simulink model "EE382lab51"  (R2016a)
settings: Solver=VariableStepAuto  StartTime=0.0  StopTime=1.0  RelTol=1e-3
settings Model: Creator=Tryrant  LastModifiedBy=Tryrant

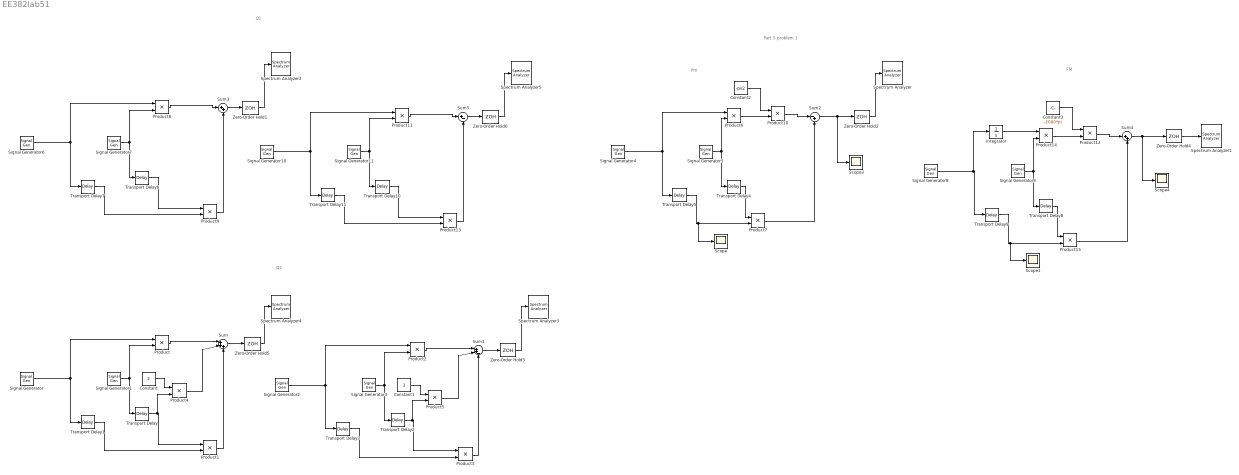
== system EE382lab51 ==
  note: Part 5 problem 1
  note: Q2
  note: Q1
  note: FM
  note: Pm
  Constant : Constant  Value=2
  Constant1 : Constant  Value=2
  Constant2 : Constant  Value=-pi/2
  Constant3 : Constant  Value=-2000*pi
  Integrator : Integrator
  Product{,1..15} (16 alike) : Product
  Scope{,1,3..4} (4 alike) : Scope
  Signal Generator{,1..3,6..7,10..11} (8 alike) : SignalGenerator  Frequency=10000
  Signal Generator4 : SignalGenerator  WaveForm=sawtooth  Frequency=1000
  Signal Generator5 : SignalGenerator  Amplitude=2  Frequency=2*pi*10^6
  Signal Generator8 : SignalGenerator  WaveForm=sawtooth  Frequency=1000
  Signal Generator9 : SignalGenerator  Amplitude=2  Frequency=2*pi*10^6  Units=rad/sec
  Spectrum Analyzer{,1..5} (6 alike) : SpectrumAnalyzer
  Sum : Sum  Inputs=|+++
  Sum1 : Sum  Inputs=|++-
  Sum2 : Sum  Inputs=|-+
  Sum3 : Sum  Inputs=|++
  Sum4 : Sum  Inputs=|++
  Sum5 : Sum  Inputs=|+-
  Transport Delay{,1..3,6..7,10..11} (8 alike) : TransportDelay  DelayTime=1/(4*10000)  BufferSize=4026
  Transport Delay4 : TransportDelay  DelayTime=1/(4*2*pi*10^6)  BufferSize=4026
  Transport Delay5 : TransportDelay  DelayTime=1/(4*1000)  BufferSize=4026
  Transport Delay8 : TransportDelay  DelayTime=1/(4*2*pi*10^6)  BufferSize=4026
  Transport Delay9 : TransportDelay  DelayTime=1/(4*1000)  BufferSize=4026
  Zero-Order Hold{1..6} (6 alike) : ZeroOrderHold  SampleTime=1/400000
  wires:
  Signal Generator1/1 -> Product/2, Transport Delay/1
  Signal Generator/1 -> Product/1, Transport Delay1/1
  Transport Delay/1 -> Product4/2, Product1/1
  Transport Delay1/1 -> Product1/2
  Product/1 -> Sum/1
  Product1/1 -> Sum/3
  Constant/1 -> Product4/1
  Product4/1 -> Sum/2
  Sum2/1 -> Scope3/1, Zero-Order Hold2/1
  Signal Generator5/1 -> Product6/2, Transport Delay4/1
  Signal Generator4/1 -> Product6/1, Transport Delay5/1
  Transport Delay4/1 -> Product7/1
  Transport Delay5/1 -> Scope/1, Product7/2
  Product10/1 -> Sum2/1
  Product6/1 -> Product10/2
  Constant2/1 -> Product10/1
  Sum4/1 -> Scope4/1, Zero-Order Hold4/1
  Signal Generator9/1 -> Product14/2, Transport Delay8/1
  Signal Generator8/1 -> Integrator/1, Transport Delay9/1
  Transport Delay8/1 -> Product15/1
  Transport Delay9/1 -> Scope1/1, Product15/2
  Product12/1 -> Sum4/1
  Product14/1 -> Product12/2
  Constant3/1 -> Product12/1
  Product7/1 -> Sum2/2
  Product15/1 -> Sum4/2
  Integrator/1 -> Product14/1
  Zero-Order Hold2/1 -> Spectrum Analyzer/1
  Zero-Order Hold4/1 -> Spectrum Analyzer1/1
  Signal Generator3/1 -> Product2/2, Transport Delay2/1
  Signal Generator2/1 -> Product2/1, Transport Delay3/1
  Transport Delay2/1 -> Product5/2, Product3/1
  Transport Delay3/1 -> Product3/2
  Product2/1 -> Sum1/1
  Product3/1 -> Sum1/3
  Constant1/1 -> Product5/1
  Product5/1 -> Sum1/2
  Signal Generator7/1 -> Product8/2, Transport Delay6/1
  Signal Generator6/1 -> Product8/1, Transport Delay7/1
  Transport Delay6/1 -> Product9/1
  Transport Delay7/1 -> Product9/2
  Product8/1 -> Sum3/1
  Product9/1 -> Sum3/2
  Sum3/1 -> Zero-Order Hold1/1
  Zero-Order Hold1/1 -> Spectrum Analyzer2/1
  Sum1/1 -> Zero-Order Hold3/1
  Zero-Order Hold3/1 -> Spectrum Analyzer3/1
  Sum/1 -> Zero-Order Hold5/1
  Zero-Order Hold5/1 -> Spectrum Analyzer4/1
  Signal Generator11/1 -> Product11/2, Transport Delay10/1
  Signal Generator10/1 -> Product11/1, Transport Delay11/1
  Transport Delay10/1 -> Product13/1
  Transport Delay11/1 -> Product13/2
  Product11/1 -> Sum5/1
  Product13/1 -> Sum5/2
  Sum5/1 -> Zero-Order Hold6/1
  Zero-Order Hold6/1 -> Spectrum Analyzer5/1
